simulink model "mode_changer"  (R2020a)
settings: Solver=FixedStepAuto  StartTime=0.0  StopTime=inf  FixedStep=0.2  RelTol=1e-3
libraries: robotlib x3
settings Model: EnablePacing=on  Creator=ivory  LastModifiedBy=ivory
settings OptimizationCC: EnhancedBackFolding=on  PassReuseOutputArgsAs=Individual arguments  ZeroExternalMemoryAtStartup=off  ZeroInternalMemoryAtStartup=off  MaxStackSize=64  OptimizeBlockOrder=speed  DifferentSizesBufferReuse=on  OptimizationCustomize=off  EfficientTunableParamExpr=on
settings DebuggingCC: ParameterTunabilityLossMsg=error
settings HardwareCC: ProdBitPerPointer=32  ProdBitPerSizeT=32  ProdBitPerPtrDiffT=32  ProdLargestAtomicFloat=None  ProdIntDivRoundTo=Undefined  ProdEndianess=Unspecified  ProdWordSize=32  ProdHWDeviceType=Generic->Unspecified (assume 32-bit Generic)
settings SFSimCC: MATLABDynamicMemAlloc=off
settings RTWCC: SystemTargetFile=ert.tlc  HardwareBoard=Robot Operating System (ROS)  TemplateMakefile=ert_default_tmf  GenerateReport=on  Toolchain=Catkin  LaunchReport=on  TargetLang=C++  GenerateWebview=on
settings CodeAppCC: ForceParamTrailComments=on  IgnoreCustomStorageClasses=off  OperatorAnnotations=on  SimulinkDataObjDesc=on  SFDataObjDesc=on  InsertBlockDesc=on

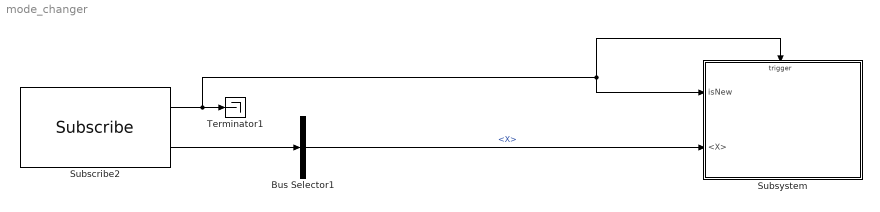
== system mode_changer ==
  Bus Selector1 : BusSelector  DialogController=Simulink.DDGSource_BusSelector  OutputSignals=Linear.X
  Subscribe2 : robotlib/Subscribe  topicSource=Specify your own  topic=/highbeams  messageType=geometry_msgs/Twist  sampleTime=-1  messageQueueLength=1
  Subsystem : Subsystem
  Terminator1 : Terminator
  wires:
  Subscribe2/2 -> Bus Selector1/1
  Subscribe2/1 -> Subsystem/Trigger, Subsystem/1(isNew), Terminator1/1
  Bus Selector1/1 -> Subsystem/2(<X>)  "<X>"

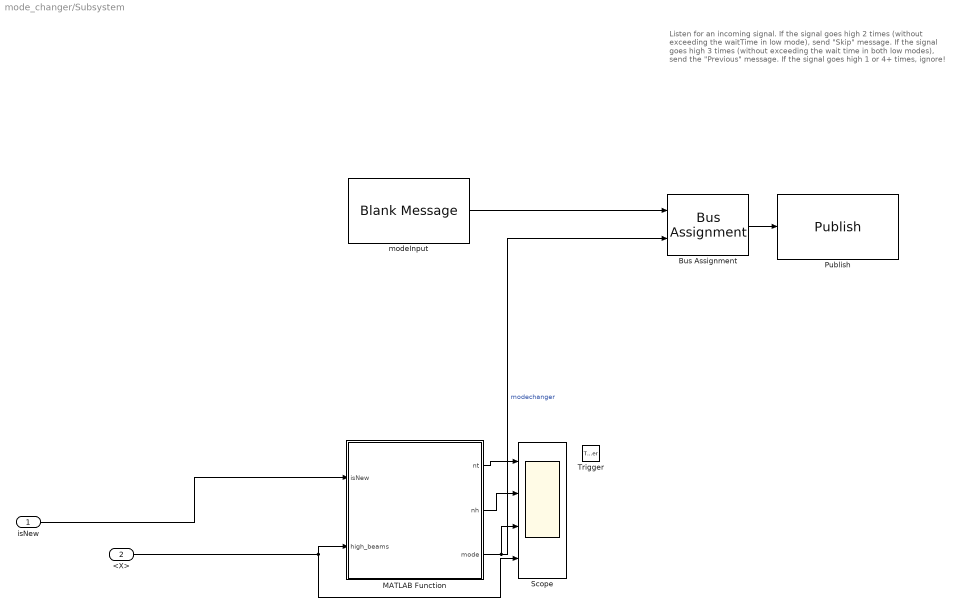
== system mode_changer/Subsystem ==
  note: Listen for an incoming signal.
      | If the signal goes high 2 times (without exceeding the waitTime in low mode), send "Skip" message. If the signal goes high 3 times (without exceeding the wait time in both low modes), send the "Previous" message. If the signal goes high 1 or 4+ times, ignore!
  isNew : Inport
  <X> : Inport  Port=2
  Trigger : TriggerPort  VariantControl=Variant  PortDimensions=1
  Bus Assignment : BusAssignment  AssignedSignals=Data
  MATLAB Function : MATLAB Function  TreatAsAtomicUnit=on
  Publish : robotlib/Publish  topicSource=Specify your own  topic=/modeChanger  messageType=std_msgs/Int8  messageQueueLength=1
  Scope : Scope  NumInputPorts=4
  modeInput : robotlib/Blank Message  messageClass=Message  entityType=std_msgs/Int8  messageType=std_msgs/Int8  SampleTime=-1
  wires:
  MATLAB Function/1(nt) -> Scope/1
  <X>/1 -> Scope/4, MATLAB Function/2(high_beams)
  isNew/1 -> MATLAB Function/1(isNew)
  MATLAB Function/2(nh) -> Scope/2
  Bus Assignment/1 -> Publish/1
  MATLAB Function/3(mode) -> Bus Assignment/2, Scope/3  "modechanger"
  modeInput/1 -> Bus Assignment/1

== matlab function mode_changer/Subsystem/MATLAB Function ==
  data: isNew input; high_beams input; nt output; nh output; mode output
function [nt, nh, mode]   = mode_changer_func(isNew, high_beams)

persistent n_toggle
persistent n_high
persistent previous


if isempty(n_toggle)
    n_toggle = 0;
    n_high = 0;
    previous = high_beams;
end

if isNew
    
    %if highbeams is low
    if high_beams == 0
        if previous == 1 && n_high < 4
            n_toggle = n_toggle + 1;
        elseif previous == 0
            n_toggle = 0;
        end
        n_high = 0;
    elseif high_beams == 1
            n_high = n_high + 1;

    end

    previous = high_beams;


    nt = n_toggle;
    nh = n_high;

    if n_toggle == 2
        mode = int8(1);
    elseif n_toggle == 3
        mode = int8(-1);
    else
        mode = int8(0);
    end
    
else
    nt = n_toggle;
    nh = n_high;
    mode = int8(0);
end
